simulink model "Roadsense_LidarPerception"  (R2025b)
settings: Solver=FixedStepDiscrete  StartTime=0.0  StopTime=0.1  FixedStep=RsTsBase  RelTol=1e-3
undefined symbols (not defined in the file or in its folder): RsGridResolution, RsGridXLimits, RsGridYLimits, RsTsLidarPerception
settings Model: DataDictionary=Roadsense_Data.sldd  Creator=ragur  LastModifiedBy=ragur

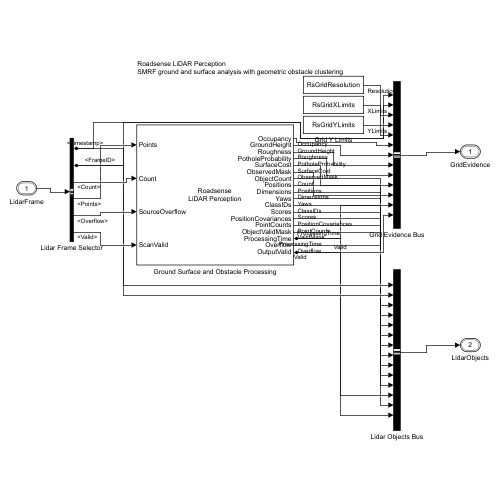
[thumbnail: Simulink's stored preview of the top-level diagram]
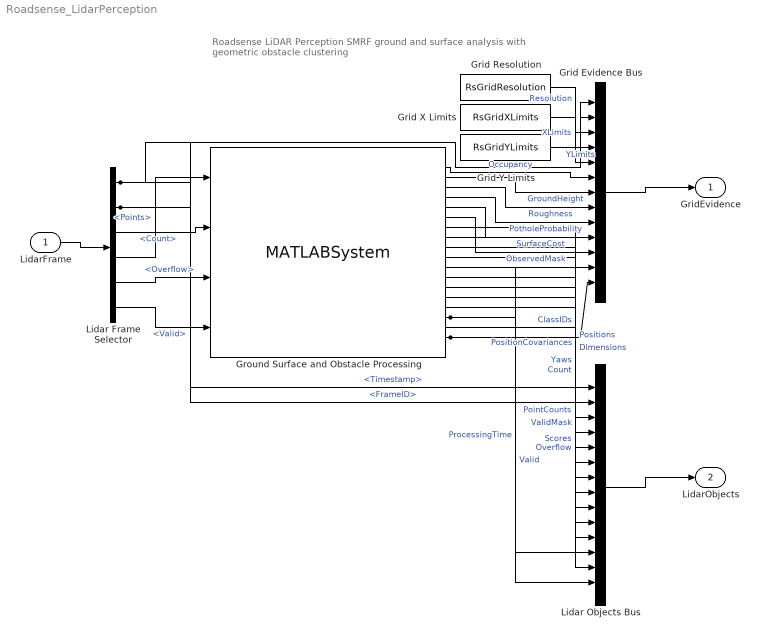
== system Roadsense_LidarPerception ==
  note: Roadsense LiDAR Perception
      | SMRF ground and surface analysis with geometric obstacle clustering
  LidarFrame : Inport  OutDataTypeStr=Bus: RsLidarFrameBus  PortDimensions=1  SampleTime=RsTsLidarPerception
  Grid Evidence Bus : BusCreator  Inputs=13  OutDataTypeStr=Bus: RsLidarGridEvidenceBus
  Grid Resolution : Constant  Value=RsGridResolution  OutDataTypeStr=single
  Grid X Limits : Constant  Value=RsGridXLimits  OutDataTypeStr=single
  Grid Y Limits : Constant  Value=RsGridYLimits  OutDataTypeStr=single
  Ground Surface and Obstacle Processing : MATLABSystem  System=RoadsenseLidarPerceptionSystem  GridResolution=single(0.25)  GridXLimits=single([-20;60])  GridYLimits=single([-25;25])  ZLimits=single([-3;5])  SMRFResolution=single(0.5)  SMRFSlopeThreshold=single(0.200000002980232)  SMRFElevationThreshold=single(0.300000011920929)  ClusterDistance=single(0.75)  MinimumClusterPoints=uint16(8)  MaximumClusterPoints=uint32(20000)  PotholeDepthThreshold=single(0.0799999982118607)  RoughnessThreshold=single(0.0500000007450581)  SimulateUsing=Interpreted execution
      mask Type: RoadsenseLidarPerceptionSystem
  Lidar Frame Selector : BusSelector  OutputSignals=Timestamp,FrameID,Count,Points,Overflow,Valid
  Lidar Objects Bus : BusCreator  Inputs=14  OutDataTypeStr=Bus: RsLidarObjectListBus
  GridEvidence : Outport  OutDataTypeStr=Bus: RsLidarGridEvidenceBus
  LidarObjects : Outport  Port=2  OutDataTypeStr=Bus: RsLidarObjectListBus
  wires:
  LidarFrame/1 -> Lidar Frame Selector/1
  Lidar Frame Selector/4 -> Ground Surface and Obstacle Processing/1  "<Points>"
  Lidar Frame Selector/3 -> Ground Surface and Obstacle Processing/2  "<Count>"
  Lidar Frame Selector/5 -> Ground Surface and Obstacle Processing/3  "<Overflow>"
  Lidar Frame Selector/6 -> Ground Surface and Obstacle Processing/4  "<Valid>"
  Lidar Frame Selector/1 -> Grid Evidence Bus/1, Lidar Objects Bus/1  "<Timestamp>"
  Lidar Frame Selector/2 -> Grid Evidence Bus/2, Lidar Objects Bus/2  "<FrameID>"
  Grid Resolution/1 -> Grid Evidence Bus/3  "Resolution"
  Grid X Limits/1 -> Grid Evidence Bus/4  "XLimits"
  Grid Y Limits/1 -> Grid Evidence Bus/5  "YLimits"
  Ground Surface and Obstacle Processing/1 -> Grid Evidence Bus/6  "Occupancy"
  Ground Surface and Obstacle Processing/2 -> Grid Evidence Bus/7  "GroundHeight"
  Ground Surface and Obstacle Processing/3 -> Grid Evidence Bus/8  "Roughness"
  Ground Surface and Obstacle Processing/4 -> Grid Evidence Bus/9  "PotholeProbability"
  Ground Surface and Obstacle Processing/5 -> Grid Evidence Bus/10  "SurfaceCost"
  Ground Surface and Obstacle Processing/6 -> Grid Evidence Bus/11  "ObservedMask"
  Ground Surface and Obstacle Processing/16 -> Grid Evidence Bus/12, Lidar Objects Bus/12  "ProcessingTime"
  Ground Surface and Obstacle Processing/18 -> Grid Evidence Bus/13, Lidar Objects Bus/14  "Valid"
  Ground Surface and Obstacle Processing/7 -> Lidar Objects Bus/3  "Count"
  Ground Surface and Obstacle Processing/8 -> Lidar Objects Bus/4  "Positions"
  Ground Surface and Obstacle Processing/9 -> Lidar Objects Bus/5  "Dimensions"
  Ground Surface and Obstacle Processing/10 -> Lidar Objects Bus/6  "Yaws"
  Ground Surface and Obstacle Processing/11 -> Lidar Objects Bus/7  "ClassIDs"
  Ground Surface and Obstacle Processing/12 -> Lidar Objects Bus/8  "Scores"
  Ground Surface and Obstacle Processing/13 -> Lidar Objects Bus/9  "PositionCovariances"
  Ground Surface and Obstacle Processing/14 -> Lidar Objects Bus/10  "PointCounts"
  Ground Surface and Obstacle Processing/15 -> Lidar Objects Bus/11  "ValidMask"
  Ground Surface and Obstacle Processing/17 -> Lidar Objects Bus/13  "Overflow"
  Grid Evidence Bus/1 -> GridEvidence/1
  Lidar Objects Bus/1 -> LidarObjects/1
